simulink model "modele_cheville"  (R2015b)
settings: Solver=ode45  StartTime=0.0  StopTime=10.0  RelTol=1e-3
PreLoadFcn:
  | cheville
undefined symbols (not defined in the file): f, Jeq, ke, ki, kred, L, R
libraries: simulink x1
settings Model: Creator=pt_ptsi  LastModifiedBy=pt_ptsi
settings DataIOCC: SaveFormat=Array
settings DebuggingCC: UnderspecifiedInitializationDetection=Classic  MergeDetectMultiDrivingBlocksExec=none  SolverPrmCheckMsg=warning  StateNameClashWarn=warning
settings HardwareCC: ProdBitPerPointer=32  ProdLargestAtomicFloat=None  ProdIntDivRoundTo=Undefined  ProdEndianess=Unspecified  ProdWordSize=32  ProdHWDeviceType=32-bit Generic
settings GRTTargetCC: GeneratePreprocessorConditionals=Disable all
settings ConfigComp: CovModelRefEnable=Off

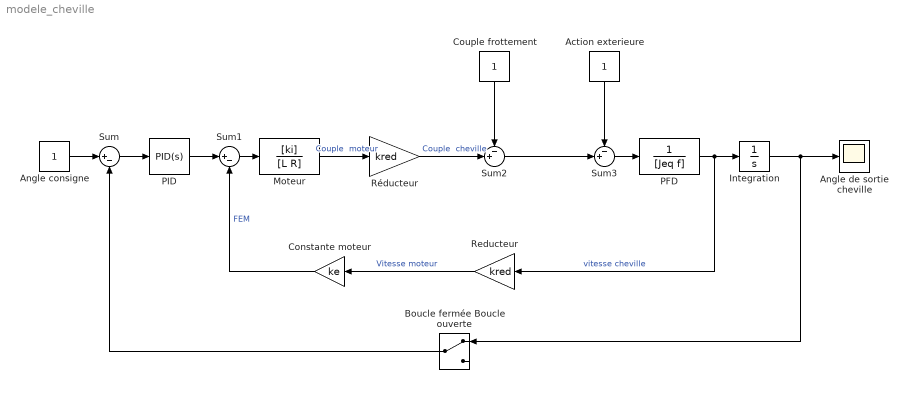
== system modele_cheville ==
  Action exterieure : Constant
  Angle consigne : Constant
  Angle de sortie cheville : Scope
  Boucle fermée Boucle ouverte : ManualSwitch
  Constante moteur : Gain  Gain=ke
  Couple frottement : Constant
  Integration : Integrator
  Moteur : TransferFcn  Numerator=[ki]  Denominator=[L R]
  PFD : TransferFcn  Denominator=[Jeq f]
  "PID " : simulink/Continuous/PID Controller  Controller=PID  TimeDomain=Continuous-time  SampleTime=-1  IntegratorMethod=Forward Euler  FilterMethod=Forward Euler  Form=Parallel  UseFilter=on  ControllerParametersSource=internal  P=1  I=1  D=0  N=100  InitialConditionSource=internal  InitialConditionForIntegrator=0  InitialConditionForFilter=0  ExternalReset=none  LimitOutput=off  UpperSaturationLimit=inf  LowerSaturationLimit=-inf  LinearizeAsGain=on  AntiWindupMode=none  Kb=1  TrackingMode=off  Kt=1  PParamMin=[]  PParamMax=[]  IParamMin=[]  IParamMax=[]  DParamMin=[]  DParamMax=[]  NParamMin=[]  NParamMax=[]  KbParamMin=[]  KbParamMax=[]  KtParamMin=[]  KtParamMax=[]  POutMin=[]  POutMax=[]  IOutMin=[]  IOutMax=[]  DOutMin=[]  DOutMax=[]  NOutMin=[]  NOutMax=[]  KbOutMin=[]  KbOutMax=[]  KtOutMin=[]  KtOutMax=[]  IntegratorOutMin=[]  IntegratorOutMax=[]  FilterOutMin=[]  FilterOutMax=[]  SumOutMin=[]  SumOutMax=[]  SumI1OutMin=[]  SumI1OutMax=[]  SumI2OutMin=[]  SumI2OutMax=[]  SumI3OutMin=[]  SumI3OutMax=[]  SumDOutMin=[]  SumDOutMax=[]  SaturationOutMin=[]  SaturationOutMax=[]  IntegratorContinuousStateAttributes=''  IntegratorStateMustResolveToSignalObject=off  IntegratorRTWStateStorageClass=Auto  FilterContinuousStateAttributes=''  FilterStateMustResolveToSignalObject=off  FilterRTWStateStorageClass=Auto  DifferentiatorICPrevScaledInput=0  DifferentiatorOutMin=[]  DifferentiatorOutMax=[]
  Reducteur : Gain  Gain=kred
  Réducteur : Gain  Gain=kred
  Sum : Sum  Inputs=|+-
  Sum1 : Sum  Inputs=|+-
  Sum2 : Sum  Inputs=-+|
  Sum3 : Sum  Inputs=-+|
  wires:
  Angle consigne/1 -> Sum/1
  Sum/1 -> "PID "/1
  "PID "/1 -> Sum1/1
  Sum1/1 -> Moteur/1
  Moteur/1 -> Réducteur/1  "Couple  moteur"
  Réducteur/1 -> Sum2/2  "Couple  cheville"
  Sum2/1 -> Sum3/2
  Sum3/1 -> PFD/1
  Couple frottement/1 -> Sum2/1
  Action exterieure/1 -> Sum3/1
  Constante moteur/1 -> Sum1/2  "FEM"
  Reducteur/1 -> Constante moteur/1  "Vitesse moteur"
  PFD/1 -> Reducteur/1, Integration/1  "vitesse cheville"
  Integration/1 -> Angle de sortie cheville/1, Boucle fermée Boucle ouverte/1
  Boucle fermée Boucle ouverte/1 -> Sum/2
